simulink model "notLinearWithControllers"  (R2019a)
settings: Solver=VariableStepAuto  StartTime=0.0  StopTime=1000  RelTol=1e-3
values from neighbouring files (symbols this model uses):
  Ka = 4.3    [q1.m]
  m = 1230    [q1.m]
  Vnom = 40/3.6    (= 11.1111111111)    [q1.m]
  Vw = 5    [q1.m]
libraries: cstblocks x3
settings Model: Creator=Nir Lalum  LastModifiedBy=Nir Lalum

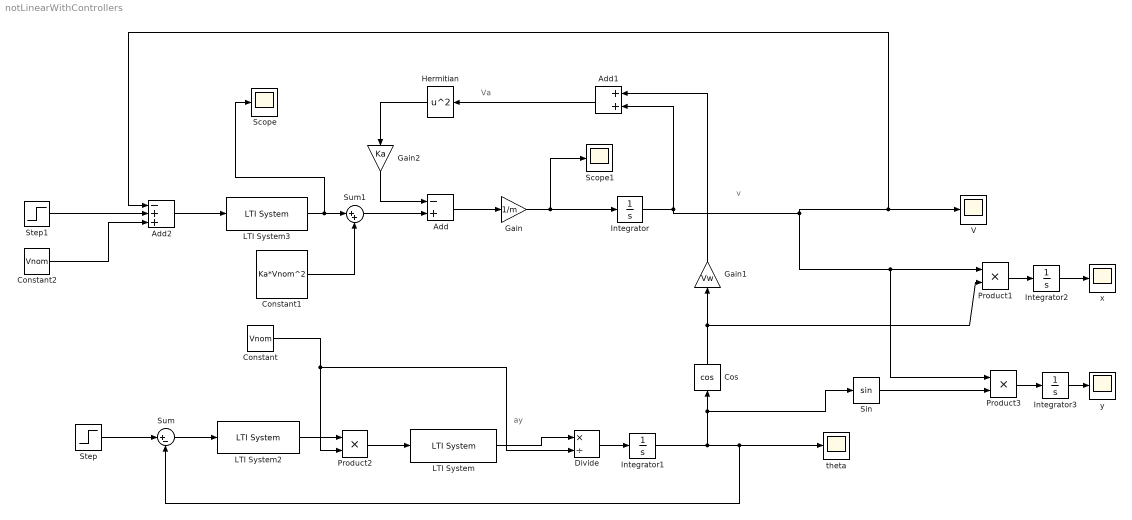
== system notLinearWithControllers ==
  note: ay
  note: v
  note: Va
  Add : Sum  Inputs=-+
  Add1 : Sum
  Add2 : Sum  Inputs=-++
  Constant : Constant  Value=Vnom
  Constant1 : Constant  Value=Ka*Vnom^2
  Constant2 : Constant  Value=Vnom
  Cos : Trigonometry  Operator=cos
  Divide : Product  Inputs=*/
  Gain : Gain  Gain=1/m
  Gain1 : Gain  Gain=Vw
  Gain2 : Gain  Gain=Ka
  Hermitian : Math  Operator=square  SaturateOnIntegerOverflow=on
  Integrator : Integrator  InitialCondition=40/3.6  LimitOutput=on  UpperSaturationLimit=90/3.6  LowerSaturationLimit=30/3.6
  Integrator1 : Integrator
  Integrator2 : Integrator
  Integrator3 : Integrator
  LTI System : cstblocks/LTI System  sys=G_ayr_ay  IC=[]
  LTI System2 : cstblocks/LTI System  sys=C_theta_tilda  IC=[]
  LTI System3 : cstblocks/LTI System  sys=C_v  IC=[]
  Product1 : Product
  Product2 : Product
  Product3 : Product
  Scope : Scope
  Scope1 : Scope
  Sin : Trigonometry
  Step : Step  Time=50  After=pi  SampleTime=0
  Step1 : Step  Time=0  After=10/3.6  SampleTime=0
  Sum : Sum  Inputs=|+-
  Sum1 : Sum  Inputs=|++
  V : Scope
  theta : Scope
  x : Scope
  y : Scope
  wires:
  Gain/1 -> Scope1/1, Integrator/1
  LTI System/1 -> Divide/1
  Divide/1 -> Integrator1/1
  Add1/1 -> Hermitian/1
  Add/1 -> Gain/1
  Cos/1 -> Product1/2, Gain1/1
  Gain1/1 -> Add1/1
  Gain2/1 -> Add/1
  Integrator1/1 -> Sin/1, Cos/1, theta/1, Sum/2
  Hermitian/1 -> Gain2/1
  Add2/1 -> LTI System3/1
  Step1/1 -> Add2/2
  Step/1 -> Sum/1
  Sum/1 -> LTI System2/1
  LTI System2/1 -> Product2/1
  Product2/1 -> LTI System/1
  Integrator/1 -> Add2/1, V/1, Product3/1, Product1/1, Add1/2
  Constant2/1 -> Add2/3
  Sin/1 -> Product3/2
  Product1/1 -> Integrator2/1
  Integrator2/1 -> x/1
  Product3/1 -> Integrator3/1
  Integrator3/1 -> y/1
  Constant/1 -> Divide/2, Product2/2
  Sum1/1 -> Add/2
  Constant1/1 -> Sum1/2
  LTI System3/1 -> Scope/1, Sum1/1
